simulink model "SWC_HALOUT_type"  (R2021b)
settings: Solver=FixedStepDiscrete  StartTime=0.0  StopTime=10.0  FixedStep=0.005  RelTol=1e-3
undefined symbols (not defined in the file): DIDLen_APPD, DIDLen_APPE, DIDLen_APPPedalZP, DIDLen_APSFunConfig, DIDLen_AutoLock, DIDLen_AutoWipHSpdEN, DIDLen_CALID, DIDLen_CDEODT, DIDLen_CLRDIST, DIDLen_DKCBLESta, DIDLen_DKCKey, DIDLen_DKCSta, DIDLen_DoorNFCAnchorSta, DIDLen_DRLDis, DIDLen_DynoMode, DIDLen_ECUNAME, DIDLen_FDDKCCoordXY, DIDLen_FMHTimer, DIDLen_LFLowPresThre, DIDLen_LFSensorID, DIDLen_LIDAAnchorSta, DIDLen_LRLowPresThre, DIDLen_LRSensorID, DIDLen_MILDIST, DIDLen_NUMPSATRIPSFLTMEMCLR, DIDLen_NVMPedalZP, DIDLen_OBDReq, DIDLen_ODOMETER, DIDLen_PKE, DIDLen_ProtocolId, DIDLen_PSA, DIDLen_QTYPSATRIPS, DIDLen_RFLowPresThre, DIDLen_RFSensorID, DIDLen_RRLowPresThre, DIDLen_RRSensorID, DIDLen_RUNTM, DIDLen_SensorMode, DIDLen_TestGroup, DIDLen_TireSize, DIDLen_TPMSLearnSta, DIDLen_TurnLampFLThreCurr, DIDLen_TurnLampFRThreCurr, DIDLen_TurnLampRLThreCurr, DIDLen_TurnLampRRThreCurr, DIDLen_UIDSta, DIDLen_USSConfig, DIDLen_UWBAnchorSta, DIDLen_VIN, DIDLen_VSS, DIDLen_WhlPres, DIDLen_WhlSensorBattSta, DIDLen_WhlTmp, DIDLen_WipRLSCmdCutFilter, DIDLen_WipRLSCmdHoldFilter, DIDLen_XWDMode, DIDNum_APPD, DIDNum_APPE, DIDNum_APPPedalZP, DIDNum_APSFunConfig ... (+504)
libraries: simulink x893, FVT_lib x320, hdlsllib x6, hcu_lib x5, halout x1
(part 5 of 11)

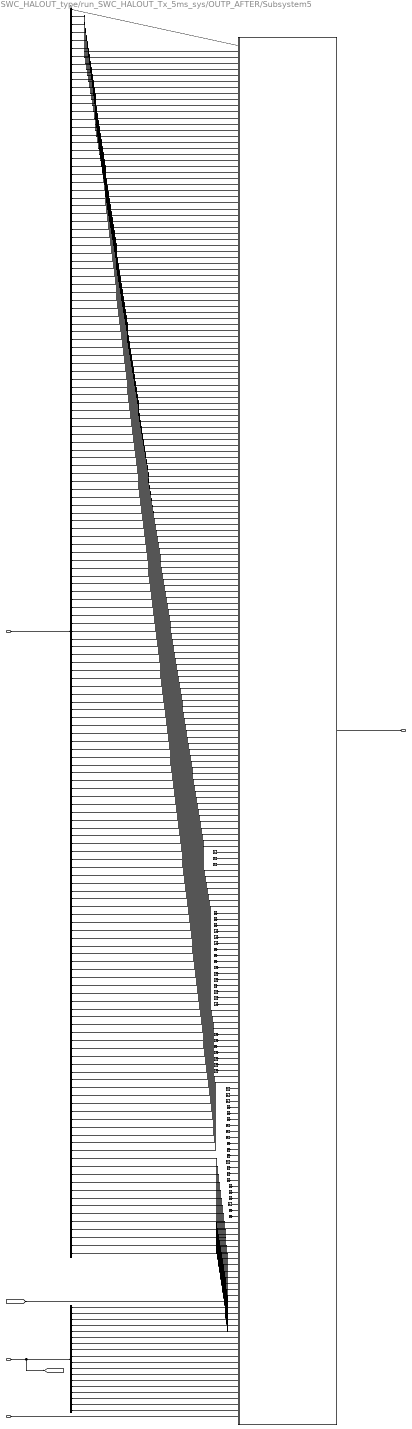
== system SWC_HALOUT_type/run_SWC_HALOUT_Tx_5ms_sys/OUTP_AFTER/Subsystem5 ==
  BOUTP_outputs : Inport
  BHAL_SYS_outputs : Inport  Port=2
  BHAL_DIDGetData_raw : Inport  Port=3
  Bus Selector : BusSelector  OutputSignals=VOUTP_AntitheftSta_enum,VOUTP_DrivetrainSelect_enum,VOUTP_WriteChkLFID_raw,VOUTP_WriteChkRFID_raw,VOUTP_WriteChkLRID_raw,VOUTP_WriteChkRRID_raw,VOUTP_WriteChkfinLFID_raw,VOUTP_WriteChkfinRFID_raw,VOUTP_WriteChkfinLRID_raw,VOUTP_WriteChkfinRRID_raw,VOUTP_LFSensorFail_flg,VOUTP_RFSensorFail_flg,VOUTP_LRSensorFail_flg,VOUTP_RRSensorFail_flg,VOUTP_LFWheelPSW_raw8,VOUTP_RFWheelPSW_raw8,VOUTP_LRWheelPSW_raw8,VOUTP_RRWheelPSW_raw8,VOUTP_LFPindi_enum,VOUTP_RFPind_enum,VOUTP_LRPindi_enum,VOUTP_RRPindi_enum,VOUTP_LFP20_raw8,VOUTP_RFP20_raw8,VOUTP_LRP20_raw8,VOUTP_RRP20_raw8,VOUTP_LFWheelPress_raw8,VOUTP_RFWheelPress_raw8,VOUTP_LRWheelPress_raw8,VOUTP_RRWheelPress_raw8,VOUTP_LFWheelTemp_C,VOUTP_RFWheelTemp_C,VOUTP_LRWheelTemp_C,VOUTP_RRWheelTemp_C,VOUTP_Flashchkdatavalid_enum,VOUTP_Flashdatavalid_enum,VOUTP_unlearnSfali_flg,VOUTP_unlearnSfailvalid_enum,VOUTP_Prepresstempvalid_enum,VOUTP_FlashS1ID_raw,VOUTP_FlashS2ID_raw,VOUTP_FlashS3ID_raw,VOUTP_FlashS4ID_raw,VOUTP_FlashIDvalid_enum,VOUTP_ACModeMem_enum,VOUTP_Face_flg,VOUTP_Foot_flg,VOUTP_Frost_flg,VOUTP_FaceM_flg,VOUTP_FootM_flg,VOUTP_CCUSyncSts_flg,VOUTP_ACForceOFF_flg,VOUTP_sigRecircSt_flg,VOUTP_RecAutoFlg_flg,VOUTP_AirIntenZone1M_enum,VOUTP_fdefog_flg,VOUTP_sigSetTempZon1St_C,VOUTP_sigSetTempZon2StM_C,VOUTP_CountAlarm_enum,VOUTP_MFSWTri_flg,VOUTP_MirrorFlodPos_flg,VOUTP_FuelDoorPos_flg,VOUTP_LockSettingStaMem_enum,VOUTP_MFRDNBrightReq_pct,VOUTP_RmLpModeENMem_enum,VOUTP_WiperFixMode_flg,VOUTP_SPTGENFunMem_enum,VOUTP_EAPS1MIN_pct,VOUTP_EAPS2MIN_pct,VOUTP_HoodSW_flg,VOUTP_TailgateSW_flg,VOUTP_CTDLockSW_flg,VOUTP_TailgateHDSW_flg,VOUTP_APMDoorControlSta_flg,VOUTP_fUnlockSingle_flg,VOUTP_SaveRegenMode_enum,VOUTP_AmbFunENFlash_enum,VOUTP_AmbWelENFlash_enum,VOUTP_AmbDimENFlash_enum,VOUTP_AmbLinkDriStaFlash_enum,VOUTP_AmbPwrWarnENFlash_enum,VOUTP_AmbODAENFlash_enum,VOUTP_AmbColorSta1_enum,VOUTP_AmbColorSta2_enum,VOUTP_AmbColorSta3_enum,VOUTP_AmbColorSta4_enum,VOUTP_AmbColorSta5_enum,VOUTP_AmbColorSta7_enum,VOUTP_AmbBrightnessSta1_enum,VOUTP_AmbBrightnessSta2_enum,VOUTP_AmbBrightnessSta3_enum,VOUTP_AmbBrightnessSta4_enum,VOUTP_AmbBrightnessSta5_enum,VOUTP_AmbBrightnessSta7_enum,VOUTP_TurnSwTimeSetSta123_enum,VOUTP_TurnSwTimeSetSta457_enum,VOUTP_FDCTHCAirIntZ3Sta_enum,VOUTP_FDCTHCREVentModeSta_enum,VOUTP_FDCTHCLEVentModeSta_enum,VOUTP_FDCTHCLEVentZSta_enum,VOUTP_FDCTHCCLEVentZSta_enum,VOUTP_FDCTHCREVentZSta_enum,VOUTP_FDCTHCCREVentZSta_enum,VOUTP_LVentEN_flg,VOUTP_FDCTHCLEVentYSta_enum,VOUTP_CLVentEN_flg,VOUTP_FDCTHCCLEVentYSta_enum,VOUTP_RVentEN_flg,VOUTP_FDCTHCREVentYSta_enum,VOUTP_CRVentEN_flg,VOUTP_FDCTHCCREVentYSta_enum,VOUTP_FDCFGSAirIntSta_enum,VOUTP_FDCFGSChSta_enum,VOUTP_FDCFGSIONSWSta_flg,VOUTP_WalkOutLkENMem_enum,VOUTP_WalkInUnLkENMem_enum,VOUTP_FollowMeENMem_enum,VOUTP_PTGUserHeight1_cnt,VOUTP_PTGUserHeight2_cnt,VOUTP_PTGUserHeight3_cnt,VOUTP_PTGUserHeight4_cnt,VOUTP_PTGUserHeight5_cnt,VOUTP_PTGUserHeight7_cnt,VOUTP_PTGOpenHeight12_enum,VOUTP_PTGOpenHeight34_enum,VOUTP_PTGOpenHeight57_enum,VOUTP_ACCLevelMem12_enum,VOUTP_ACCLevelMem34_enum,VOUTP_ACCLevelMem57_enum,VOUTP_AutoLockMem_enum,VOUTP_AutoUnlockMem_enum,VOUTP_MILDIST_km,VOUTP_CLRDIST_km,VOUTP_NUMPSATRIPSFLTMEMCLR_cnt,VOUTP_PSAR_sec,VOUTP_PSAL_sec,VOUTP_IPSAR_sec,VOUTP_IPSAL_sec,VOUTP_CPSAR_sec,VOUTP_CPSAL_sec,VOUTP_PKERNumerator_kphsqr,VOUTP_PKELNumerator_kphsqr,VOUTP_ODOMETER_km,VOUTP_ResetCDEODTR_km,VOUTP_QTYPSATRIPSR_cnt,VOUTP_QTYPSATRIPSL_cnt,VOUTP_HMIKey1FuncSta_enum,VOUTP_HMIKey2FuncSta_enum,VOUTP_HMIKey3FuncSta_enum,VOUTP_HMIKey4FuncSta_enum,VOUTP_HMIKey5FuncSta_enum,VOUTP_HMIKey6FuncSta_enum,VOUTP_HMIKey7FuncSta_enum,VOUTP_HMIKey8FuncSta_enum,VOUTP_AutoWipHSpdENSta_flg,VOUTP_ModelVersion_raw,VOUTP_ModelVersionChksum_raw,VOUTP_DIDModelVersion_raw,VOUTP_DIDModelVersionChksum_raw
  Bus Selector1 : BusSelector  OutputSignals=VHAL_RandomnumberY_raw1,VHAL_RandomnumberY_raw2,VHAL_RandomnumberY_raw3,VHAL_RandomnumberY_raw4,VHAL_RandomnumberY_raw5,VHAL_RandomnumberY_raw6,VHAL_RandomnumberY_raw7,VHAL_RandomnumberY_raw8,VHAL_funAuto_flg,VHAL_DiagDRLOFF_flg,VHAL_DiagFMHT_s,VHAL_DiagFLTC_mA,VHAL_DiagFRTC_mA,VHAL_DiagRLTC_mA,VHAL_DiagRRTC_mA,VHAL_USSConfig_raw8,VHAL_TireSize_raw8,VHAL_APSFunConfig_raw8
  Enabled Subsystem : Subsystem  TreatAsAtomicUnit=on
  Ground{,1..47} (48 alike) : Ground
  HAL_NvmWriteData_raw : Outport
  wires:
  BOUTP_outputs/1 -> Bus Selector/1
  Enabled Subsystem/1(HAL_NvmWriteData_raw) -> HAL_NvmWriteData_raw/1
  Bus Selector1/2 -> Enabled Subsystem/210(VHAL_RandomnumberY_raw2)  "<VHAL_RandomnumberY_raw2>"
  Bus Selector1/3 -> Enabled Subsystem/211(VHAL_RandomnumberY_raw3)  "<VHAL_RandomnumberY_raw3>"
  Bus Selector1/4 -> Enabled Subsystem/212(VHAL_RandomnumberY_raw4)  "<VHAL_RandomnumberY_raw4>"
  Bus Selector1/5 -> Enabled Subsystem/213(VHAL_RandomnumberY_raw5)  "<VHAL_RandomnumberY_raw5>"
  Bus Selector1/6 -> Enabled Subsystem/214(VHAL_RandomnumberY_raw6)  "<VHAL_RandomnumberY_raw6>"
  Bus Selector1/7 -> Enabled Subsystem/215(VHAL_RandomnumberY_raw7)  "<VHAL_RandomnumberY_raw7>"
  Bus Selector1/8 -> Enabled Subsystem/216(VHAL_RandomnumberY_raw8)  "<VHAL_RandomnumberY_raw8>"
  Bus Selector/24 -> Enabled Subsystem/24(VOUTP_RFP20_raw8)  "<VOUTP_RFP20_raw8>"
  Bus Selector/23 -> Enabled Subsystem/23(VOUTP_LFP20_raw8)  "<VOUTP_LFP20_raw8>"
  Bus Selector/25 -> Enabled Subsystem/25(VOUTP_LRP20_raw8)  "<VOUTP_LRP20_raw8>"
  Bus Selector/22 -> Enabled Subsystem/22(VOUTP_RRPindi_enum)  "<VOUTP_RRPindi_enum>"
  Bus Selector/26 -> Enabled Subsystem/26(VOUTP_RRP20_raw8)  "<VOUTP_RRP20_raw8>"
  Bus Selector/21 -> Enabled Subsystem/21(VOUTP_LRPindi_enum)  "<VOUTP_LRPindi_enum>"
  Bus Selector/27 -> Enabled Subsystem/27(VOUTP_LFWheelPress_raw8)  "<VOUTP_LFWheelPress_raw8>"
  Bus Selector/20 -> Enabled Subsystem/20(VOUTP_RFPindi_enum)  "<VOUTP_RFPind_enum>"
  Bus Selector/28 -> Enabled Subsystem/28(VOUTP_RFWheelPress_raw8)  "<VOUTP_RFWheelPress_raw8>"
  Bus Selector/19 -> Enabled Subsystem/19(VOUTP_LFPindi_enum)  "<VOUTP_LFPindi_enum>"
  Bus Selector/29 -> Enabled Subsystem/29(VOUTP_LRWheelPress_raw8)  "<VOUTP_LRWheelPress_raw8>"
  Bus Selector/56 -> Enabled Subsystem/56(VOUTP_fdefog_flg)  "<VOUTP_fdefog_flg>"
  Bus Selector/18 -> Enabled Subsystem/18(VOUTP_RRWheelPSW_raw8)  "<VOUTP_RRWheelPSW_raw8>"
  Bus Selector/30 -> Enabled Subsystem/30(VOUTP_RRWheelPress_raw8)  "<VOUTP_RRWheelPress_raw8>"
  Bus Selector/55 -> Enabled Subsystem/55(VOUTP_AirIntenZone1M_enum)  "<VOUTP_AirIntenZone1M_enum>"
  Bus Selector/17 -> Enabled Subsystem/17(VOUTP_LRWheelPSW_raw8)  "<VOUTP_LRWheelPSW_raw8>"
  Bus Selector/31 -> Enabled Subsystem/31(VOUTP_LFWheelTemp_C)  "<VOUTP_LFWheelTemp_C>"
  Bus Selector/54 -> Enabled Subsystem/54(VOUTP_RecAutoFlg_flg)  "<VOUTP_RecAutoFlg_flg>"
  Bus Selector/16 -> Enabled Subsystem/16(VOUTP_RFWheelPSW_raw8)  "<VOUTP_RFWheelPSW_raw8>"
  Bus Selector/32 -> Enabled Subsystem/32(VOUTP_RFWheelTemp_C)  "<VOUTP_RFWheelTemp_C>"
  Bus Selector/53 -> Enabled Subsystem/53(VOUTP_sigRecircSt_flg)  "<VOUTP_sigRecircSt_flg>"
  Bus Selector/15 -> Enabled Subsystem/15(VOUTP_LFWheelPSW_raw8)  "<VOUTP_LFWheelPSW_raw8>"
  Bus Selector/33 -> Enabled Subsystem/33(VOUTP_LRWheelTemp_C)  "<VOUTP_LRWheelTemp_C>"
  Bus Selector/52 -> Enabled Subsystem/52(VOUTP_ACForceOFF_flg)  "<VOUTP_ACForceOFF_flg>"
  Bus Selector/14 -> Enabled Subsystem/14(VOUTP_RRSensorFail_flg)  "<VOUTP_RRSensorFail_flg>"
  Bus Selector/34 -> Enabled Subsystem/34(VOUTP_RRWheelTemp_C)  "<VOUTP_RRWheelTemp_C>"
  Bus Selector/51 -> Enabled Subsystem/51(VOUTP_CCUSyncSts_flg)  "<VOUTP_CCUSyncSts_flg>"
  Bus Selector/13 -> Enabled Subsystem/13(VOUTP_LRSensorFail_flg)  "<VOUTP_LRSensorFail_flg>"
  Bus Selector/35 -> Enabled Subsystem/35(VOUTP_Flashchkdatavalid_enum)  "<VOUTP_Flashchkdatavalid_enum>"
  Bus Selector/50 -> Enabled Subsystem/50(VOUTP_FootM_flg)  "<VOUTP_FootM_flg>"
  Bus Selector/12 -> Enabled Subsystem/12(VOUTP_RFSensorFail_flg)  "<VOUTP_RFSensorFail_flg>"
  Bus Selector/36 -> Enabled Subsystem/36(VOUTP_Flashdatavalid_enum)  "<VOUTP_Flashdatavalid_enum>"
  Bus Selector/49 -> Enabled Subsystem/49(VOUTP_FaceM_flg)  "<VOUTP_FaceM_flg>"
  Bus Selector/11 -> Enabled Subsystem/11(VOUTP_LFSensorFail_flg)  "<VOUTP_LFSensorFail_flg>"
  Bus Selector/37 -> Enabled Subsystem/37(VOUTP_unlearnSfali_flg)  "<VOUTP_unlearnSfali_flg>"
  Bus Selector/48 -> Enabled Subsystem/48(VOUTP_Frost_flg)  "<VOUTP_Frost_flg>"
  Bus Selector/38 -> Enabled Subsystem/38(VOUTP_unlearnSfailvalid_enum)  "<VOUTP_unlearnSfailvalid_enum>"
  Bus Selector/47 -> Enabled Subsystem/47(VOUTP_Foot_flg)  "<VOUTP_Foot_flg>"
  Bus Selector/39 -> Enabled Subsystem/39(VOUTP_Prepresstempvalid_enum)  "<VOUTP_Prepresstempvalid_enum>"
  Bus Selector/46 -> Enabled Subsystem/46(VOUTP_Face_flg)  "<VOUTP_Face_flg>"
  Bus Selector/2 -> Enabled Subsystem/2(VOUTP_DrivetrainSelect_enum)  "<VOUTP_DrivetrainSelect_enum>"
  Bus Selector/1 -> Enabled Subsystem/1(VOUTP_AntitheftSta_enum)  "<VOUTP_AntitheftSta_enum>"
  Bus Selector/10 -> Enabled Subsystem/10(VOUTP_WriteChkfinRRID_raw)  "<VOUTP_WriteChkfinRRID_raw>"
  Bus Selector/9 -> Enabled Subsystem/9(VOUTP_WriteChkfinLRID_raw)  "<VOUTP_WriteChkfinLRID_raw>"
  Bus Selector/8 -> Enabled Subsystem/8(VOUTP_WriteChkfinRFID_raw)  "<VOUTP_WriteChkfinRFID_raw>"
  Bus Selector/7 -> Enabled Subsystem/7(VOUTP_WriteChkfinLFID_raw)  "<VOUTP_WriteChkfinLFID_raw>"
  Bus Selector/6 -> Enabled Subsystem/6(VOUTP_WriteChkRRID_raw)  "<VOUTP_WriteChkRRID_raw>"
  Bus Selector/5 -> Enabled Subsystem/5(VOUTP_WriteChkLRID_raw)  "<VOUTP_WriteChkLRID_raw>"
  Bus Selector/4 -> Enabled Subsystem/4(VOUTP_WriteChkRFID_raw)  "<VOUTP_WriteChkRFID_raw>"
  Bus Selector/3 -> Enabled Subsystem/3(VOUTP_WriteChkLFID_raw)  "<VOUTP_WriteChkLFID_raw>"
  Bus Selector/58 -> Enabled Subsystem/58(VOUTP_sigSetTempZon2StM_C)  "<VOUTP_sigSetTempZon2StM_C>"
  Bus Selector/59 -> Enabled Subsystem/59(VOUT_CountAlarm_enum)  "<VOUTP_CountAlarm_enum>"
  Bus Selector/57 -> Enabled Subsystem/57(VOUTP_sigSetTempZon1St_C)  "<VOUTP_sigSetTempZon1St_C>"
  Bus Selector/60 -> Enabled Subsystem/60(VOUTP_MFSWTri_flg)  "<VOUTP_MFSWTri_flg>"
  Bus Selector/61 -> Enabled Subsystem/61(VOUTP_MirrorFlodPos_flg)  "<VOUTP_MirrorFlodPos_flg>"
  Bus Selector/62 -> Enabled Subsystem/62(VOUTP_FuelDoorPos_flg)  "<VOUTP_FuelDoorPos_flg>"
  Bus Selector/63 -> Enabled Subsystem/63(VOUTP_LockSetting_flg)  "<VOUTP_LockSettingStaMem_enum>"
  Bus Selector/64 -> Enabled Subsystem/64(VOUTP_MFRDNBrightReq_pct)  "<VOUTP_MFRDNBrightReq_pct>"
  Bus Selector/65 -> Enabled Subsystem/65(VOUTP_RoomLampMode_flg)  "<VOUTP_RmLpModeENMem_enum>"
  Bus Selector/66 -> Enabled Subsystem/66(VOUTP_WiperFixMode_flg)  "<VOUTP_WiperFixMode_flg>"
  Bus Selector/67 -> Enabled Subsystem/67(VOUTP_IVIPTGUSStaSW_flg)  "<VOUTP_SPTGENFunMem_enum>"
  Bus Selector1/1 -> Enabled Subsystem/209(VHAL_RandomnumberY_raw1)  "<VHAL_RandomnumberY_raw1>"
  Bus Selector/45 -> Enabled Subsystem/45(VOUTP_ACModeMem_enum)  "<VOUTP_ACModeMem_enum>"
  Bus Selector/40 -> Enabled Subsystem/40(VOUTP_FlashS1ID_raw)  "<VOUTP_FlashS1ID_raw>"
  Bus Selector/41 -> Enabled Subsystem/41(VOUTP_FlashS2ID_raw)  "<VOUTP_FlashS2ID_raw>"
  Bus Selector/42 -> Enabled Subsystem/42(VOUTP_FlashS3ID_raw)  "<VOUTP_FlashS3ID_raw>"
  Bus Selector/43 -> Enabled Subsystem/43(VOUTP_FlashS41ID_raw)  "<VOUTP_FlashS4ID_raw>"
  Bus Selector/44 -> Enabled Subsystem/44(VOUTP_FlashIDvalid_enum)  "<VOUTP_FlashIDvalid_enum>"
  BHAL_SYS_outputs/1 -> [BHAL_SYS_outputs], Bus Selector1/1
  Bus Selector/68 -> Enabled Subsystem/68(VOUTP_EAPS1MIN_pct)  "<VOUTP_EAPS1MIN_pct>"
  Bus Selector/69 -> Enabled Subsystem/69(VOUTP_EAPS2MIN_pct)  "<VOUTP_EAPS2MIN_pct>"
  Bus Selector/70 -> Enabled Subsystem/70(VOUTP_HoodSW_flg)  "<VOUTP_HoodSW_flg>"
  Bus Selector/71 -> Enabled Subsystem/71(VOUTP_TailgateSW_flg)  "<VOUTP_TailgateSW_flg>"
  Bus Selector/72 -> Enabled Subsystem/72(VOUTP_CTDLockSW_flg)  "<VOUTP_CTDLockSW_flg>"
  Bus Selector/73 -> Enabled Subsystem/73(VOUTP_TailgateHDSW_flg)  "<VOUTP_TailgateHDSW_flg>"
  Bus Selector/74 -> Enabled Subsystem/74(VOUTP_APMDoorControlSta_flg)  "<VOUTP_APMDoorControlSta_flg>"
  Bus Selector1/9 -> Enabled Subsystem/217(VHAL_funAuto_flg)  "<VHAL_funAuto_flg>"
  Bus Selector1/10 -> Enabled Subsystem/218(VHAL_DiagDRLOFF_flg)  "<VHAL_DiagDRLOFF_flg>"
  Bus Selector1/11 -> Enabled Subsystem/219(VHAL_DiagFMHT_s)  "<VHAL_DiagFMHT_s>"
  Bus Selector1/12 -> Enabled Subsystem/220(VHAL_DiagFLTC_mA)  "<VHAL_DiagFLTC_mA>"
  Bus Selector1/13 -> Enabled Subsystem/221(VHAL_DiagFRTC_mA)  "<VHAL_DiagFRTC_mA>"
  Bus Selector1/14 -> Enabled Subsystem/222(VHAL_DiagRLTC_mA)  "<VHAL_DiagRLTC_mA>"
  Bus Selector1/15 -> Enabled Subsystem/223(VHAL_DiagRRTC_mA)  "<VHAL_DiagRRTC_mA>"
  Bus Selector1/16 -> Enabled Subsystem/224(VHAL_USSConfig_raw8)  "<VHAL_USSConfig_raw8>"
  Bus Selector1/17 -> Enabled Subsystem/225(VHAL_TireSize_raw8)  "<VHAL_TireSize_raw8>"
  Bus Selector1/18 -> Enabled Subsystem/226(VHAL_APSFunConfig_raw8)  "<VHAL_APSFunConfig_raw8>"
  Bus Selector/75 -> Enabled Subsystem/75(VOUTP_fUnlockSingle_flg)  "<VOUTP_fUnlockSingle_flg>"
  Bus Selector/76 -> Enabled Subsystem/76(VOUTP_SaveRegenMode_enum)  "<VOUTP_SaveRegenMode_enum>"
  Bus Selector/77 -> Enabled Subsystem/77(VOUTP_AmbFunENFlash_enum)  "<VOUTP_AmbFunENFlash_enum>"
  Bus Selector/78 -> Enabled Subsystem/78(VOUTP_AmbWelENFlash_enum)  "<VOUTP_AmbWelENFlash_enum>"
  Bus Selector/79 -> Enabled Subsystem/79(VOUTP_AmbDimENFlash_enum)  "<VOUTP_AmbDimENFlash_enum>"
  Bus Selector/80 -> Enabled Subsystem/80(VOUTP_AmbLinkDriStaFlash_enum)  "<VOUTP_AmbLinkDriStaFlash_enum>"
  Bus Selector/81 -> Enabled Subsystem/81(VOUTP_AmbPwrWarnENFlash_enum)  "<VOUTP_AmbPwrWarnENFlash_enum>"
  Bus Selector/82 -> Enabled Subsystem/82(VOUTP_AmbODAENFlash_enum)  "<VOUTP_AmbODAENFlash_enum>"
  Bus Selector/83 -> Enabled Subsystem/83(VOUTP_AmbColorSta1_enum)  "<VOUTP_AmbColorSta1_enum>"
  Bus Selector/84 -> Enabled Subsystem/84(VOUTP_AmbColorSta2_enum)  "<VOUTP_AmbColorSta2_enum>"
  Bus Selector/85 -> Enabled Subsystem/85(VOUTP_AmbColorSta3_enum)  "<VOUTP_AmbColorSta3_enum>"
  Bus Selector/86 -> Enabled Subsystem/86(VOUTP_AmbColorSta4_enum)  "<VOUTP_AmbColorSta4_enum>"
  Bus Selector/87 -> Enabled Subsystem/87(VOUTP_AmbColorSta5_enum)  "<VOUTP_AmbColorSta5_enum>"
  Bus Selector/88 -> Enabled Subsystem/88(VOUTP_AmbColorSta7_enum)  "<VOUTP_AmbColorSta7_enum>"
  Bus Selector/89 -> Enabled Subsystem/89(VOUTP_AmbBrightnessSta1_enum)  "<VOUTP_AmbBrightnessSta1_enum>"
  Bus Selector/90 -> Enabled Subsystem/90(VOUTP_AmbBrightnessSta2_enum)  "<VOUTP_AmbBrightnessSta2_enum>"
  Bus Selector/91 -> Enabled Subsystem/91(VOUTP_AmbBrightnessSta3_enum)  "<VOUTP_AmbBrightnessSta3_enum>"
  Bus Selector/92 -> Enabled Subsystem/92(VOUTP_AmbBrightnessSta4_enum)  "<VOUTP_AmbBrightnessSta4_enum>"
  Bus Selector/93 -> Enabled Subsystem/93(VOUTP_AmbBrightnessSta5_enum)  "<VOUTP_AmbBrightnessSta5_enum>"
  Bus Selector/94 -> Enabled Subsystem/94(VOUTP_AmbBrightnessSta7_enum)  "<VOUTP_AmbBrightnessSta7_enum>"
  Bus Selector/95 -> Enabled Subsystem/95(VOUTP_TurnSwTimeSetSta123_enum)  "<VOUTP_TurnSwTimeSetSta123_enum>"
  Bus Selector/96 -> Enabled Subsystem/96(VOUTP_TurnSwTimeSetSta457_enum)  "<VOUTP_TurnSwTimeSetSta457_enum>"
  Bus Selector/97 -> Enabled Subsystem/97(VOUTP_FDCTHCAirIntZ3Sta_enum)  "<VOUTP_FDCTHCAirIntZ3Sta_enum>"
  Bus Selector/98 -> Enabled Subsystem/98(VOUTP_FDCTHCREVentModeSta_enum)  "<VOUTP_FDCTHCREVentModeSta_enum>"
  Bus Selector/99 -> Enabled Subsystem/99(VOUTP_FDCTHCLEVentModeSta_enum)  "<VOUTP_FDCTHCLEVentModeSta_enum>"
  Bus Selector/100 -> Enabled Subsystem/100(VOUTP_FDCTHCLEVentZSta_enum)  "<VOUTP_FDCTHCLEVentZSta_enum>"
  Bus Selector/101 -> Enabled Subsystem/101(VOUTP_FDCTHCCLEVentZSta_enum)  "<VOUTP_FDCTHCCLEVentZSta_enum>"
  Bus Selector/102 -> Enabled Subsystem/102(VOUTP_FDCTHCREVentZSta_enum)  "<VOUTP_FDCTHCREVentZSta_enum>"
  Bus Selector/103 -> Enabled Subsystem/103(VOUTP_FDCTHCCREVentZSta_enum)  "<VOUTP_FDCTHCCREVentZSta_enum>"
  Bus Selector/104 -> Enabled Subsystem/104(VOUTP_LVentEN_flg)  "<VOUTP_LVentEN_flg>"
  Bus Selector/105 -> Enabled Subsystem/105(VOUTP_FDCTHCLEVentYSta_enum)  "<VOUTP_FDCTHCLEVentYSta_enum>"
  Bus Selector/106 -> Enabled Subsystem/106(VOUTP_CLVentEN_flg)  "<VOUTP_CLVentEN_flg>"
  Bus Selector/107 -> Enabled Subsystem/107(VOUTP_FDCTHCCLEVentYSta_enum)  "<VOUTP_FDCTHCCLEVentYSta_enum>"
  Bus Selector/108 -> Enabled Subsystem/108(VOUTP_RVentEN_flg)  "<VOUTP_RVentEN_flg>"
  Bus Selector/109 -> Enabled Subsystem/109(VOUTP_FDCTHCREVentYSta_enum)  "<VOUTP_FDCTHCREVentYSta_enum>"
  Bus Selector/110 -> Enabled Subsystem/110(VOUTP_CRVentEN_flg)  "<VOUTP_CRVentEN_flg>"
  Bus Selector/111 -> Enabled Subsystem/111(VOUTP_FDCTHCCREVentYSta_enum)  "<VOUTP_FDCTHCCREVentYSta_enum>"
  Bus Selector/112 -> Enabled Subsystem/112(VOUTP_FDCFGSAirIntSta_enum)  "<VOUTP_FDCFGSAirIntSta_enum>"
  Bus Selector/113 -> Enabled Subsystem/113(VOUTP_FDCFGSChSta_enum)  "<VOUTP_FDCFGSChSta_enum>"
  Bus Selector/114 -> Enabled Subsystem/114(VOUTP_FDCFGSIONSWSta_flg)  "<VOUTP_FDCFGSIONSWSta_flg>"
  Bus Selector/115 -> Enabled Subsystem/115(VOUTP_WalkOutLkENFunSta_flg)  "<VOUTP_WalkOutLkENMem_enum>"
  Bus Selector/116 -> Enabled Subsystem/116(VOUTP_WalkInUnLkENFunSta_flg)  "<VOUTP_WalkInUnLkENMem_enum>"
  Bus Selector/117 -> Enabled Subsystem/117(VOUTP_FollowMeENFunSta_flg)  "<VOUTP_FollowMeENMem_enum>"
  Bus Selector/118 -> Enabled Subsystem/118(VOUTP_PTGUserHeight1_cnt)  "<VOUTP_PTGUserHeight1_cnt>"
  Bus Selector/119 -> Enabled Subsystem/119(VOUTP_PTGUserHeight2_cnt)  "<VOUTP_PTGUserHeight2_cnt>"
  Bus Selector/120 -> Enabled Subsystem/120(VOUTP_PTGUserHeight3_cnt)  "<VOUTP_PTGUserHeight3_cnt>"
  Bus Selector/121 -> Enabled Subsystem/121(VOUTP_PTGUserHeight4_cnt)  "<VOUTP_PTGUserHeight4_cnt>"
  Bus Selector/122 -> Enabled Subsystem/122(VOUTP_PTGUserHeight5_cnt)  "<VOUTP_PTGUserHeight5_cnt>"
  Bus Selector/123 -> Enabled Subsystem/123(VOUTP_PTGUserHeight7_cnt)  "<VOUTP_PTGUserHeight7_cnt>"
  Bus Selector/124 -> Enabled Subsystem/124(VOUTP_PTGOpenHeight12_enum)  "<VOUTP_PTGOpenHeight12_enum>"
  Bus Selector/125 -> Enabled Subsystem/125(VOUTP_PTGOpenHeight34_enum)  "<VOUTP_PTGOpenHeight34_enum>"
  Bus Selector/126 -> Enabled Subsystem/126(VOUTP_PTGOpenHeight57_enum)  "<VOUTP_PTGOpenHeight57_enum>"
  BHAL_DIDGetData_raw/1 -> Enabled Subsystem/227(BHAL_DIDGetData_raw)
  Bus Selector/127 -> Enabled Subsystem/127(VOUTP_ACCLevelMem12_enum)  "<VOUTP_ACCLevelMem12_enum>"
  Bus Selector/128 -> Enabled Subsystem/128(VOUTP_ACCLevelMem34_enum)  "<VOUTP_ACCLevelMem34_enum>"
  Bus Selector/129 -> Enabled Subsystem/129(VOUTP_ACCLevelMem57_enum)  "<VOUTP_ACCLevelMem57_enum>"
  Bus Selector/130 -> Enabled Subsystem/130(VOUTP_AutoLockMem_enum)  "<VOUTP_AutoLockMem_enum>"
  Bus Selector/131 -> Enabled Subsystem/131(VOUTP_AutoUnlockMem_enum)  "<VOUTP_AutoUnlockMem_enum>"
  Bus Selector/132 -> Enabled Subsystem/132(VOUTP_MILDIST_km)  "<VOUTP_MILDIST_km>"
  Bus Selector/133 -> Enabled Subsystem/133(VOUTP_CLRDIST_km)  "<VOUTP_CLRDIST_km>"
  Bus Selector/134 -> Enabled Subsystem/137(VOUTP_NUMPSATRIPSFLTMEMCLR_cnt)  "<VOUTP_NUMPSATRIPSFLTMEMCLR_cnt>"
  Bus Selector/135 -> Enabled Subsystem/138(VOUTP_PSAR_sec)  "<VOUTP_PSAR_sec>"
  Bus Selector/136 -> Enabled Subsystem/139(VOUTP_PSAL_sec)  "<VOUTP_PSAL_sec>"
  Bus Selector/137 -> Enabled Subsystem/140(VOUTP_IPSAR_sec)  "<VOUTP_IPSAR_sec>"
  Bus Selector/138 -> Enabled Subsystem/141(VOUTP_IPSAL_sec)  "<VOUTP_IPSAL_sec>"
  Bus Selector/139 -> Enabled Subsystem/142(VOUTP_CPSAR_sec)  "<VOUTP_CPSAR_sec>"
  Bus Selector/140 -> Enabled Subsystem/143(VOUTP_CPSAL_sec)  "<VOUTP_CPSAL_sec>"
  Bus Selector/143 -> Enabled Subsystem/162(VOUTP_ODOMETER_km)  "<VOUTP_ODOMETER_km>"
  Bus Selector/145 -> Enabled Subsystem/171(VOUTP_QTYPSATRIPSR_cnt)  "<VOUTP_QTYPSATRIPSR_cnt>"
  Bus Selector/146 -> Enabled Subsystem/172(VOUTP_QTYPSATRIPSL_cnt)  "<VOUTP_QTYPSATRIPSL_cnt>"
  Bus Selector/144 -> Enabled Subsystem/163(VOUTP_ResetCDEODTR_km)  "<VOUTP_ResetCDEODTR_km>"
  Bus Selector/141 -> Enabled Subsystem/160(VOUTP_PKERNumerator_kphsqr)  "<VOUTP_PKERNumerator_kphsqr>"
  Bus Selector/142 -> Enabled Subsystem/161(VOUTP_PKELNumerator_kphsqr)  "<VOUTP_PKELNumerator_kphsqr>"
  [BHAL_SYS_outputs] -> Enabled Subsystem/208(BHAL_SYS_outputs)
  Bus Selector/147 -> Enabled Subsystem/195(VOUTP_HMIKey1FuncSta_enum)  "<VOUTP_HMIKey1FuncSta_enum>"
  Bus Selector/148 -> Enabled Subsystem/196(VOUTP_HMIKey2FuncSta_enum)  "<VOUTP_HMIKey2FuncSta_enum>"
  Bus Selector/149 -> Enabled Subsystem/197(VOUTP_HMIKey3FuncSta_enum)  "<VOUTP_HMIKey3FuncSta_enum>"
  Bus Selector/150 -> Enabled Subsystem/198(VOUTP_HMIKey4FuncSta_enum)  "<VOUTP_HMIKey4FuncSta_enum>"
  Bus Selector/151 -> Enabled Subsystem/199(VOUTP_HMIKey5FuncSta_enum)  "<VOUTP_HMIKey5FuncSta_enum>"
  Bus Selector/152 -> Enabled Subsystem/200(VOUTP_HMIKey6FuncSta_enum)  "<VOUTP_HMIKey6FuncSta_enum>"
  Bus Selector/153 -> Enabled Subsystem/201(VOUTP_HMIKey7FuncSta_enum)  "<VOUTP_HMIKey7FuncSta_enum>"
  Bus Selector/154 -> Enabled Subsystem/202(VOUTP_HMIKey8FuncSta_enum)  "<VOUTP_HMIKey8FuncSta_enum>"
  Bus Selector/155 -> Enabled Subsystem/203(VOUTP_AutoWipHSpdENSta_flg)  "<VOUTP_AutoWipHSpdENSta_flg>"
  Bus Selector/156 -> Enabled Subsystem/204(VOUTP_ModelVersion_raw)  "<VOUTP_ModelVersion_raw>"
  Bus Selector/157 -> Enabled Subsystem/205(VOUTP_ModelVersionChksum_raw)  "<VOUTP_ModelVersionChksum_raw>"
  Bus Selector/158 -> Enabled Subsystem/206(VOUTP_DIDModelVersion_raw)  "<VOUTP_DIDModelVersion_raw>"
  Bus Selector/159 -> Enabled Subsystem/207(VOUTP_DIDModelVersionChksum_raw)  "<VOUTP_DIDModelVersionChksum_raw>"
  Ground/1 -> Enabled Subsystem/134(VOUTP_WARMUPS_cnt)
  Ground1/1 -> Enabled Subsystem/135(VOUTP_MILTIME_min)
  Ground2/1 -> Enabled Subsystem/136(VOUTP_CLRTIME_min)
  Ground4/1 -> Enabled Subsystem/145(VOUTP_IGNCNTR_cnt)
  Ground5/1 -> Enabled Subsystem/146(VOUTP_TNBCPSAR_Ahr)
  Ground3/1 -> Enabled Subsystem/144(VOUTP_HVBNAH_Ahr)
  Ground6/1 -> Enabled Subsystem/147(VOUTP_TNBCPSAL_Ahr)
  Ground8/1 -> Enabled Subsystem/149(VOUTP_TNECPSAL_kWh)
  Ground7/1 -> Enabled Subsystem/148(VOUTP_TNECPSAR_kWh)
  Ground13/1 -> Enabled Subsystem/154(VOUTP_GECHGOVCDCR_kWh)
  Ground14/1 -> Enabled Subsystem/155(VOUTP_GECHGOVCDCL_kWh)
  Ground12/1 -> Enabled Subsystem/153(VOUTP_TGEOVCL_kWh)
  Ground9/1 -> Enabled Subsystem/150(VOUTP_TEBPSAR_kWh)
  Ground11/1 -> Enabled Subsystem/152(VOUTP_TGEOVCR_kWh)
  Ground10/1 -> Enabled Subsystem/151(VOUTP_TEBPSAL_kWh)
  Ground15/1 -> Enabled Subsystem/156(VOUTP_GECHGOVCACR_kWh)
  Ground16/1 -> Enabled Subsystem/157(VOUTP_GECHGOVCACL_kWh)
  Ground18/1 -> Enabled Subsystem/159(VOUTP_RESSV2XENNONPSAL_kWh)
  Ground17/1 -> Enabled Subsystem/158(VOUTP_RESSV2XENNONPSAR_kWh)
  Ground19/1 -> Enabled Subsystem/164(VOUTP_AvgBattTempPSAR_C)
  Ground23/1 -> Enabled Subsystem/168(VOUTP_AvgBattTempOFFR_C)
  Ground24/1 -> Enabled Subsystem/169(VOUTP_AvgBattTempOFFL_C)
  Ground20/1 -> Enabled Subsystem/165(VOUTP_AvgBattTempPSAL_C)
  Ground22/1 -> Enabled Subsystem/167(VOUTP_AvgBattTempOVCL_C)
  Ground21/1 -> Enabled Subsystem/166(VOUTP_AvgBattTempOVCR_C)
  Ground25/1 -> Enabled Subsystem/170(VOUTP_HVBNE_kWh)
  Ground27/1 -> Enabled Subsystem/181(VOUTP_RESSTIMESOCCHGRNGR_s)
  Ground41/1 -> Enabled Subsystem/179(VOUTP_RESSTIMESOCPSARNGR_s)
  Ground26/1 -> Enabled Subsystem/180(VOUTP_RESSTIMESOCPSARNGL_s)
  Ground28/1 -> Enabled Subsystem/182(VOUTP_RESSTIMESOCOFFRNGL_s)
  Ground29/1 -> Enabled Subsystem/183(VOUTP_MAXBATTEMPL_C)
  Ground36/1 -> Enabled Subsystem/174(VOUTP_ETMBTOER_kWh)
  Ground37/1 -> Enabled Subsystem/175(VOUTP_ETMBTOEL_kWh)
  Ground34/1 -> Enabled Subsystem/188(VOUTP_AVGBATTEMPL_C)
  Ground30/1 -> Enabled Subsystem/184(VOUTP_MINBATTEMPL_C)
  Ground35/1 -> Enabled Subsystem/173(VOUTP_RESSCNTDODRNGR_cnt)
  Ground31/1 -> Enabled Subsystem/185(VOUTP_RESSTIMESOCCHGRNGL_s)
  Ground38/1 -> Enabled Subsystem/176(VOUTP_RESSCNTDODRNGL_cnt)
  Ground33/1 -> Enabled Subsystem/187(VOUTP_AVGBATTEMPL_sec)
  Ground40/1 -> Enabled Subsystem/178(VOUTP_ETMATOEL_kWh)
  Ground32/1 -> Enabled Subsystem/186(VOUTP_RESSTIMESOCOFFRNGR_s)
  Ground39/1 -> Enabled Subsystem/177(VOUTP_ETMATOER_kWh)
  Ground46/1 -> Enabled Subsystem/193(VOUTP_OFFR_sec)
  Ground47/1 -> Enabled Subsystem/194(VOUTP_OFFL_sec)
  Ground45/1 -> Enabled Subsystem/192(VOUTP_OVCL_sec)
  Ground44/1 -> Enabled Subsystem/191(VOUTP_OVCR_sec)
  Ground43/1 -> Enabled Subsystem/190(VOUTP_BattTempPSAL_sec)
  Ground42/1 -> Enabled Subsystem/189(VOUTP_BattTempPSAR_sec)

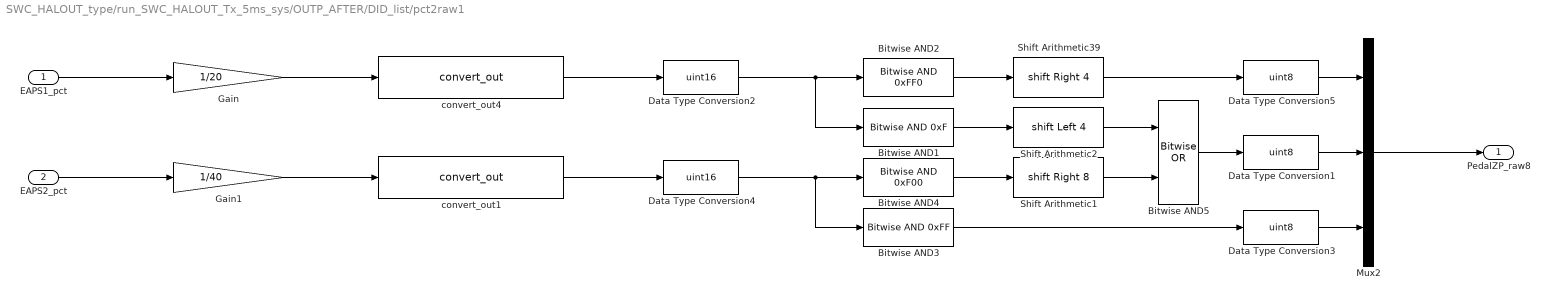
== system SWC_HALOUT_type/run_SWC_HALOUT_Tx_5ms_sys/OUTP_AFTER/DID_list/pct2raw1 ==
  EAPS1_pct : Inport
  EAPS2_pct : Inport  Port=2
  Bitwise AND1 : simulink/Logic and Bit Operations/Bitwise Operator  logicop=AND  UseBitMask=on  BitMask=0xF  BitMaskRealWorld=Stored Integer
  Bitwise AND2 : simulink/Logic and Bit Operations/Bitwise Operator  logicop=AND  UseBitMask=on  BitMask=0xFF0  BitMaskRealWorld=Stored Integer
  Bitwise AND3 : simulink/Logic and Bit Operations/Bitwise Operator  logicop=AND  UseBitMask=on  BitMask=0xFF  BitMaskRealWorld=Stored Integer
  Bitwise AND4 : simulink/Logic and Bit Operations/Bitwise Operator  logicop=AND  UseBitMask=on  BitMask=0xF00  BitMaskRealWorld=Stored Integer
  Bitwise AND5 : simulink/Logic and Bit Operations/Bitwise Operator  logicop=OR  UseBitMask=off  NumInputPorts=2  BitMask=0xFF  BitMaskRealWorld=Stored Integer
  Data Type Conversion1 : DataTypeConversion  OutDataTypeStr=uint8
  Data Type Conversion2 : DataTypeConversion  OutDataTypeStr=uint16
  Data Type Conversion3 : DataTypeConversion  OutDataTypeStr=uint8
  Data Type Conversion4 : DataTypeConversion  OutDataTypeStr=uint16
  Data Type Conversion5 : DataTypeConversion  OutDataTypeStr=uint8
  Gain : Gain  Gain=1/20
  Gain1 : Gain  Gain=1/40
  Mux2 : Mux  Inputs=3
  Shift Arithmetic1 : ArithShift  BitShiftNumber=8  BitShiftDirection=Right
  Shift Arithmetic2 : ArithShift  BitShiftNumber=4  BitShiftDirection=Left
  Shift Arithmetic39 : ArithShift  BitShiftNumber=4  BitShiftDirection=Right
  convert_out1 : FVT_lib/hal/convert_out  gain=0.001  offset=0
  convert_out4 : FVT_lib/hal/convert_out  gain=0.001  offset=0
  PedalZP_raw8 : Outport
  wires:
  Data Type Conversion1/1 -> Mux2/2
  Bitwise AND5/1 -> Data Type Conversion1/1
  Shift Arithmetic1/1 -> Bitwise AND5/2
  Shift Arithmetic2/1 -> Bitwise AND5/1
  Gain1/1 -> convert_out1/1
  Gain/1 -> convert_out4/1
  EAPS1_pct/1 -> Gain/1
  convert_out4/1 -> Data Type Conversion2/1
  convert_out1/1 -> Data Type Conversion4/1
  EAPS2_pct/1 -> Gain1/1
  Bitwise AND3/1 -> Data Type Conversion3/1
  Bitwise AND4/1 -> Shift Arithmetic1/1
  Data Type Conversion4/1 -> Bitwise AND3/1, Bitwise AND4/1
  Data Type Conversion3/1 -> Mux2/3
  Data Type Conversion5/1 -> Mux2/1
  Data Type Conversion2/1 -> Bitwise AND2/1, Bitwise AND1/1
  Bitwise AND2/1 -> Shift Arithmetic39/1
  Shift Arithmetic39/1 -> Data Type Conversion5/1
  Mux2/1 -> PedalZP_raw8/1
  Bitwise AND1/1 -> Shift Arithmetic2/1

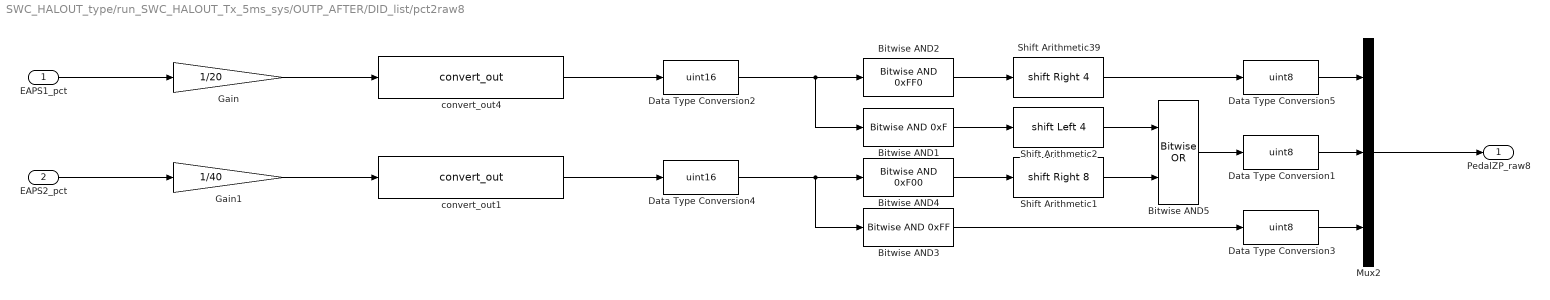
== system SWC_HALOUT_type/run_SWC_HALOUT_Tx_5ms_sys/OUTP_AFTER/DID_list/pct2raw8 ==
  EAPS1_pct : Inport
  EAPS2_pct : Inport  Port=2
  Bitwise AND1 : simulink/Logic and Bit Operations/Bitwise Operator  logicop=AND  UseBitMask=on  BitMask=0xF  BitMaskRealWorld=Stored Integer
  Bitwise AND2 : simulink/Logic and Bit Operations/Bitwise Operator  logicop=AND  UseBitMask=on  BitMask=0xFF0  BitMaskRealWorld=Stored Integer
  Bitwise AND3 : simulink/Logic and Bit Operations/Bitwise Operator  logicop=AND  UseBitMask=on  BitMask=0xFF  BitMaskRealWorld=Stored Integer
  Bitwise AND4 : simulink/Logic and Bit Operations/Bitwise Operator  logicop=AND  UseBitMask=on  BitMask=0xF00  BitMaskRealWorld=Stored Integer
  Bitwise AND5 : simulink/Logic and Bit Operations/Bitwise Operator  logicop=OR  UseBitMask=off  NumInputPorts=2  BitMask=0xFF  BitMaskRealWorld=Stored Integer
  Data Type Conversion1 : DataTypeConversion  OutDataTypeStr=uint8
  Data Type Conversion2 : DataTypeConversion  OutDataTypeStr=uint16
  Data Type Conversion3 : DataTypeConversion  OutDataTypeStr=uint8
  Data Type Conversion4 : DataTypeConversion  OutDataTypeStr=uint16
  Data Type Conversion5 : DataTypeConversion  OutDataTypeStr=uint8
  Gain : Gain  Gain=1/20
  Gain1 : Gain  Gain=1/40
  Mux2 : Mux  Inputs=3
  Shift Arithmetic1 : ArithShift  BitShiftNumber=8  BitShiftDirection=Right
  Shift Arithmetic2 : ArithShift  BitShiftNumber=4  BitShiftDirection=Left
  Shift Arithmetic39 : ArithShift  BitShiftNumber=4  BitShiftDirection=Right
  convert_out1 : FVT_lib/hal/convert_out  gain=0.001  offset=0
  convert_out4 : FVT_lib/hal/convert_out  gain=0.001  offset=0
  PedalZP_raw8 : Outport
  wires:
  Bitwise AND1/1 -> Shift Arithmetic2/1
  Mux2/1 -> PedalZP_raw8/1
  Shift Arithmetic39/1 -> Data Type Conversion5/1
  Bitwise AND2/1 -> Shift Arithmetic39/1
  Data Type Conversion2/1 -> Bitwise AND1/1, Bitwise AND2/1
  Data Type Conversion5/1 -> Mux2/1
  Data Type Conversion3/1 -> Mux2/3
  Data Type Conversion4/1 -> Bitwise AND4/1, Bitwise AND3/1
  Bitwise AND4/1 -> Shift Arithmetic1/1
  Bitwise AND3/1 -> Data Type Conversion3/1
  EAPS2_pct/1 -> Gain1/1
  convert_out1/1 -> Data Type Conversion4/1
  convert_out4/1 -> Data Type Conversion2/1
  EAPS1_pct/1 -> Gain/1
  Gain/1 -> convert_out4/1
  Gain1/1 -> convert_out1/1
  Shift Arithmetic2/1 -> Bitwise AND5/1
  Shift Arithmetic1/1 -> Bitwise AND5/2
  Bitwise AND5/1 -> Data Type Conversion1/1
  Data Type Conversion1/1 -> Mux2/2

== system SWC_HALOUT_type/run_SWC_HALOUT_Tx_5ms_sys/OUTP_AFTER/DID_list/uint16Touint8Array1 ==
  In1 : Inport
  Bitwise AND1 : simulink/Logic and Bit Operations/Bitwise Operator  logicop=AND  UseBitMask=on  BitMask=bin2dec('00000000000000000000000011111111')  BitMaskRealWorld=Stored Integer
  Bitwise AND2 : simulink/Logic and Bit Operations/Bitwise Operator  logicop=AND  UseBitMask=on  BitMask=bin2dec('00000000000000001111111100000000')  BitMaskRealWorld=Stored Integer
  Data Type Conversion1 : DataTypeConversion  OutDataTypeStr=uint8
  Data Type Conversion2 : DataTypeConversion  OutDataTypeStr=uint16
  Data Type Conversion5 : DataTypeConversion  OutDataTypeStr=uint8
  Mux2 : Mux  Inputs=2
  Shift Arithmetic39 : ArithShift  BitShiftNumber=8  BitShiftDirection=Right
  Out1 : Outport
  wires:
  Data Type Conversion1/1 -> Mux2/2
  Data Type Conversion5/1 -> Mux2/1
  Data Type Conversion2/1 -> Bitwise AND2/1, Bitwise AND1/1
  Bitwise AND2/1 -> Shift Arithmetic39/1
  Shift Arithmetic39/1 -> Data Type Conversion5/1
  In1/1 -> Data Type Conversion2/1
  Mux2/1 -> Out1/1
  Bitwise AND1/1 -> Data Type Conversion1/1

== system SWC_HALOUT_type/run_SWC_HALOUT_Tx_5ms_sys/OUTP_AFTER/DID_list/uint16Touint8Array10 ==
  In1 : Inport
  Bitwise AND1 : simulink/Logic and Bit Operations/Bitwise Operator  logicop=AND  UseBitMask=on  BitMask=bin2dec('00000000000000000000000011111111')  BitMaskRealWorld=Stored Integer
  Bitwise AND2 : simulink/Logic and Bit Operations/Bitwise Operator  logicop=AND  UseBitMask=on  BitMask=bin2dec('00000000000000001111111100000000')  BitMaskRealWorld=Stored Integer
  Data Type Conversion1 : DataTypeConversion  OutDataTypeStr=uint8
  Data Type Conversion2 : DataTypeConversion  OutDataTypeStr=uint16
  Data Type Conversion5 : DataTypeConversion  OutDataTypeStr=uint8
  Mux2 : Mux  Inputs=2
  Shift Arithmetic39 : ArithShift  BitShiftNumber=8  BitShiftDirection=Right
  Out1 : Outport
  wires:
  Data Type Conversion1/1 -> Mux2/2
  Data Type Conversion5/1 -> Mux2/1
  Data Type Conversion2/1 -> Bitwise AND2/1, Bitwise AND1/1
  Bitwise AND2/1 -> Shift Arithmetic39/1
  Shift Arithmetic39/1 -> Data Type Conversion5/1
  In1/1 -> Data Type Conversion2/1
  Mux2/1 -> Out1/1
  Bitwise AND1/1 -> Data Type Conversion1/1

== system SWC_HALOUT_type/run_SWC_HALOUT_Tx_5ms_sys/OUTP_AFTER/DID_list/uint16Touint8Array11 ==
  In1 : Inport
  Bitwise AND1 : simulink/Logic and Bit Operations/Bitwise Operator  logicop=AND  UseBitMask=on  BitMask=bin2dec('00000000000000000000000011111111')  BitMaskRealWorld=Stored Integer
  Bitwise AND2 : simulink/Logic and Bit Operations/Bitwise Operator  logicop=AND  UseBitMask=on  BitMask=bin2dec('00000000000000001111111100000000')  BitMaskRealWorld=Stored Integer
  Data Type Conversion1 : DataTypeConversion  OutDataTypeStr=uint8
  Data Type Conversion2 : DataTypeConversion  OutDataTypeStr=uint16
  Data Type Conversion5 : DataTypeConversion  OutDataTypeStr=uint8
  Mux2 : Mux  Inputs=2
  Shift Arithmetic39 : ArithShift  BitShiftNumber=8  BitShiftDirection=Right
  Out1 : Outport
  wires:
  Bitwise AND1/1 -> Data Type Conversion1/1
  Mux2/1 -> Out1/1
  In1/1 -> Data Type Conversion2/1
  Shift Arithmetic39/1 -> Data Type Conversion5/1
  Bitwise AND2/1 -> Shift Arithmetic39/1
  Data Type Conversion2/1 -> Bitwise AND1/1, Bitwise AND2/1
  Data Type Conversion5/1 -> Mux2/1
  Data Type Conversion1/1 -> Mux2/2

== system SWC_HALOUT_type/run_SWC_HALOUT_Tx_5ms_sys/OUTP_AFTER/DID_list/uint16Touint8Array12 ==
  In1 : Inport
  Bitwise AND1 : simulink/Logic and Bit Operations/Bitwise Operator  logicop=AND  UseBitMask=on  BitMask=bin2dec('00000000000000000000000011111111')  BitMaskRealWorld=Stored Integer
  Bitwise AND2 : simulink/Logic and Bit Operations/Bitwise Operator  logicop=AND  UseBitMask=on  BitMask=bin2dec('00000000000000001111111100000000')  BitMaskRealWorld=Stored Integer
  Data Type Conversion1 : DataTypeConversion  OutDataTypeStr=uint8
  Data Type Conversion2 : DataTypeConversion  OutDataTypeStr=uint16
  Data Type Conversion5 : DataTypeConversion  OutDataTypeStr=uint8
  Mux2 : Mux  Inputs=2
  Shift Arithmetic39 : ArithShift  BitShiftNumber=8  BitShiftDirection=Right
  Out1 : Outport
  wires:
  Data Type Conversion1/1 -> Mux2/2
  Data Type Conversion5/1 -> Mux2/1
  Data Type Conversion2/1 -> Bitwise AND2/1, Bitwise AND1/1
  Bitwise AND2/1 -> Shift Arithmetic39/1
  Shift Arithmetic39/1 -> Data Type Conversion5/1
  In1/1 -> Data Type Conversion2/1
  Mux2/1 -> Out1/1
  Bitwise AND1/1 -> Data Type Conversion1/1

== system SWC_HALOUT_type/run_SWC_HALOUT_Tx_5ms_sys/OUTP_AFTER/DID_list/uint16Touint8Array13 ==
  In1 : Inport
  Bitwise AND1 : simulink/Logic and Bit Operations/Bitwise Operator  logicop=AND  UseBitMask=on  BitMask=bin2dec('00000000000000000000000011111111')  BitMaskRealWorld=Stored Integer
  Bitwise AND2 : simulink/Logic and Bit Operations/Bitwise Operator  logicop=AND  UseBitMask=on  BitMask=bin2dec('00000000000000001111111100000000')  BitMaskRealWorld=Stored Integer
  Data Type Conversion1 : DataTypeConversion  OutDataTypeStr=uint8
  Data Type Conversion2 : DataTypeConversion  OutDataTypeStr=uint16
  Data Type Conversion5 : DataTypeConversion  OutDataTypeStr=uint8
  Mux2 : Mux  Inputs=2
  Shift Arithmetic39 : ArithShift  BitShiftNumber=8  BitShiftDirection=Right
  Out1 : Outport
  wires:
  Data Type Conversion1/1 -> Mux2/2
  Data Type Conversion5/1 -> Mux2/1
  Data Type Conversion2/1 -> Bitwise AND2/1, Bitwise AND1/1
  Bitwise AND2/1 -> Shift Arithmetic39/1
  Shift Arithmetic39/1 -> Data Type Conversion5/1
  In1/1 -> Data Type Conversion2/1
  Mux2/1 -> Out1/1
  Bitwise AND1/1 -> Data Type Conversion1/1

== system SWC_HALOUT_type/run_SWC_HALOUT_Tx_5ms_sys/OUTP_AFTER/DID_list/uint16Touint8Array14 ==
  In1 : Inport
  Bitwise AND1 : simulink/Logic and Bit Operations/Bitwise Operator  logicop=AND  UseBitMask=on  BitMask=bin2dec('00000000000000000000000011111111')  BitMaskRealWorld=Stored Integer
  Bitwise AND2 : simulink/Logic and Bit Operations/Bitwise Operator  logicop=AND  UseBitMask=on  BitMask=bin2dec('00000000000000001111111100000000')  BitMaskRealWorld=Stored Integer
  Data Type Conversion1 : DataTypeConversion  OutDataTypeStr=uint8
  Data Type Conversion2 : DataTypeConversion  OutDataTypeStr=uint16
  Data Type Conversion5 : DataTypeConversion  OutDataTypeStr=uint8
  Mux2 : Mux  Inputs=2
  Shift Arithmetic39 : ArithShift  BitShiftNumber=8  BitShiftDirection=Right
  Out1 : Outport
  wires:
  Bitwise AND1/1 -> Data Type Conversion1/1
  Mux2/1 -> Out1/1
  In1/1 -> Data Type Conversion2/1
  Shift Arithmetic39/1 -> Data Type Conversion5/1
  Bitwise AND2/1 -> Shift Arithmetic39/1
  Data Type Conversion2/1 -> Bitwise AND1/1, Bitwise AND2/1
  Data Type Conversion5/1 -> Mux2/1
  Data Type Conversion1/1 -> Mux2/2

== system SWC_HALOUT_type/run_SWC_HALOUT_Tx_5ms_sys/OUTP_AFTER/DID_list/uint16Touint8Array15 ==
  In1 : Inport
  Bitwise AND1 : simulink/Logic and Bit Operations/Bitwise Operator  logicop=AND  UseBitMask=on  BitMask=bin2dec('00000000000000000000000011111111')  BitMaskRealWorld=Stored Integer
  Bitwise AND2 : simulink/Logic and Bit Operations/Bitwise Operator  logicop=AND  UseBitMask=on  BitMask=bin2dec('00000000000000001111111100000000')  BitMaskRealWorld=Stored Integer
  Data Type Conversion1 : DataTypeConversion  OutDataTypeStr=uint8
  Data Type Conversion2 : DataTypeConversion  OutDataTypeStr=uint16
  Data Type Conversion5 : DataTypeConversion  OutDataTypeStr=uint8
  Mux2 : Mux  Inputs=2
  Shift Arithmetic39 : ArithShift  BitShiftNumber=8  BitShiftDirection=Right
  Out1 : Outport
  wires:
  Data Type Conversion1/1 -> Mux2/2
  Data Type Conversion5/1 -> Mux2/1
  Data Type Conversion2/1 -> Bitwise AND2/1, Bitwise AND1/1
  Bitwise AND2/1 -> Shift Arithmetic39/1
  Shift Arithmetic39/1 -> Data Type Conversion5/1
  In1/1 -> Data Type Conversion2/1
  Mux2/1 -> Out1/1
  Bitwise AND1/1 -> Data Type Conversion1/1

== system SWC_HALOUT_type/run_SWC_HALOUT_Tx_5ms_sys/OUTP_AFTER/DID_list/uint16Touint8Array16 ==
  In1 : Inport
  Bitwise AND1 : simulink/Logic and Bit Operations/Bitwise Operator  logicop=AND  UseBitMask=on  BitMask=bin2dec('00000000000000000000000011111111')  BitMaskRealWorld=Stored Integer
  Bitwise AND2 : simulink/Logic and Bit Operations/Bitwise Operator  logicop=AND  UseBitMask=on  BitMask=bin2dec('00000000000000001111111100000000')  BitMaskRealWorld=Stored Integer
  Data Type Conversion1 : DataTypeConversion  OutDataTypeStr=uint8
  Data Type Conversion2 : DataTypeConversion  OutDataTypeStr=uint16
  Data Type Conversion5 : DataTypeConversion  OutDataTypeStr=uint8
  Mux2 : Mux  Inputs=2
  Shift Arithmetic39 : ArithShift  BitShiftNumber=8  BitShiftDirection=Right
  Out1 : Outport
  wires:
  Data Type Conversion1/1 -> Mux2/2
  Data Type Conversion5/1 -> Mux2/1
  Data Type Conversion2/1 -> Bitwise AND2/1, Bitwise AND1/1
  Bitwise AND2/1 -> Shift Arithmetic39/1
  Shift Arithmetic39/1 -> Data Type Conversion5/1
  In1/1 -> Data Type Conversion2/1
  Mux2/1 -> Out1/1
  Bitwise AND1/1 -> Data Type Conversion1/1

== system SWC_HALOUT_type/run_SWC_HALOUT_Tx_5ms_sys/OUTP_AFTER/DID_list/uint16Touint8Array17 ==
  In1 : Inport
  Bitwise AND1 : simulink/Logic and Bit Operations/Bitwise Operator  logicop=AND  UseBitMask=on  BitMask=bin2dec('00000000000000000000000011111111')  BitMaskRealWorld=Stored Integer
  Bitwise AND2 : simulink/Logic and Bit Operations/Bitwise Operator  logicop=AND  UseBitMask=on  BitMask=bin2dec('00000000000000001111111100000000')  BitMaskRealWorld=Stored Integer
  Data Type Conversion1 : DataTypeConversion  OutDataTypeStr=uint8
  Data Type Conversion2 : DataTypeConversion  OutDataTypeStr=uint16
  Data Type Conversion5 : DataTypeConversion  OutDataTypeStr=uint8
  Mux2 : Mux  Inputs=2
  Shift Arithmetic39 : ArithShift  BitShiftNumber=8  BitShiftDirection=Right
  Out1 : Outport
  wires:
  Bitwise AND1/1 -> Data Type Conversion1/1
  Mux2/1 -> Out1/1
  In1/1 -> Data Type Conversion2/1
  Shift Arithmetic39/1 -> Data Type Conversion5/1
  Bitwise AND2/1 -> Shift Arithmetic39/1
  Data Type Conversion2/1 -> Bitwise AND1/1, Bitwise AND2/1
  Data Type Conversion5/1 -> Mux2/1
  Data Type Conversion1/1 -> Mux2/2

== system SWC_HALOUT_type/run_SWC_HALOUT_Tx_5ms_sys/OUTP_AFTER/DID_list/uint16Touint8Array18 ==
  In1 : Inport
  Bitwise AND1 : simulink/Logic and Bit Operations/Bitwise Operator  logicop=AND  UseBitMask=on  BitMask=bin2dec('00000000000000000000000011111111')  BitMaskRealWorld=Stored Integer
  Bitwise AND2 : simulink/Logic and Bit Operations/Bitwise Operator  logicop=AND  UseBitMask=on  BitMask=bin2dec('00000000000000001111111100000000')  BitMaskRealWorld=Stored Integer
  Data Type Conversion1 : DataTypeConversion  OutDataTypeStr=uint8
  Data Type Conversion2 : DataTypeConversion  OutDataTypeStr=uint16
  Data Type Conversion5 : DataTypeConversion  OutDataTypeStr=uint8
  Mux2 : Mux  Inputs=2
  Shift Arithmetic39 : ArithShift  BitShiftNumber=8  BitShiftDirection=Right
  Out1 : Outport
  wires:
  Data Type Conversion1/1 -> Mux2/2
  Data Type Conversion5/1 -> Mux2/1
  Data Type Conversion2/1 -> Bitwise AND2/1, Bitwise AND1/1
  Bitwise AND2/1 -> Shift Arithmetic39/1
  Shift Arithmetic39/1 -> Data Type Conversion5/1
  In1/1 -> Data Type Conversion2/1
  Mux2/1 -> Out1/1
  Bitwise AND1/1 -> Data Type Conversion1/1

== system SWC_HALOUT_type/run_SWC_HALOUT_Tx_5ms_sys/OUTP_AFTER/DID_list/uint16Touint8Array19 ==
  In1 : Inport
  Bitwise AND1 : simulink/Logic and Bit Operations/Bitwise Operator  logicop=AND  UseBitMask=on  BitMask=bin2dec('00000000000000000000000011111111')  BitMaskRealWorld=Stored Integer
  Bitwise AND2 : simulink/Logic and Bit Operations/Bitwise Operator  logicop=AND  UseBitMask=on  BitMask=bin2dec('00000000000000001111111100000000')  BitMaskRealWorld=Stored Integer
  Data Type Conversion1 : DataTypeConversion  OutDataTypeStr=uint8
  Data Type Conversion2 : DataTypeConversion  OutDataTypeStr=uint16
  Data Type Conversion5 : DataTypeConversion  OutDataTypeStr=uint8
  Mux2 : Mux  Inputs=2
  Shift Arithmetic39 : ArithShift  BitShiftNumber=8  BitShiftDirection=Right
  Out1 : Outport
  wires:
  Bitwise AND1/1 -> Data Type Conversion1/1
  Mux2/1 -> Out1/1
  In1/1 -> Data Type Conversion2/1
  Shift Arithmetic39/1 -> Data Type Conversion5/1
  Bitwise AND2/1 -> Shift Arithmetic39/1
  Data Type Conversion2/1 -> Bitwise AND1/1, Bitwise AND2/1
  Data Type Conversion5/1 -> Mux2/1
  Data Type Conversion1/1 -> Mux2/2

== system SWC_HALOUT_type/run_SWC_HALOUT_Tx_5ms_sys/OUTP_AFTER/DID_list/uint16Touint8Array2 ==
  In1 : Inport
  Bitwise AND1 : simulink/Logic and Bit Operations/Bitwise Operator  logicop=AND  UseBitMask=on  BitMask=bin2dec('00000000000000000000000011111111')  BitMaskRealWorld=Stored Integer
  Bitwise AND2 : simulink/Logic and Bit Operations/Bitwise Operator  logicop=AND  UseBitMask=on  BitMask=bin2dec('00000000000000001111111100000000')  BitMaskRealWorld=Stored Integer
  Data Type Conversion1 : DataTypeConversion  OutDataTypeStr=uint8
  Data Type Conversion2 : DataTypeConversion  OutDataTypeStr=uint16
  Data Type Conversion5 : DataTypeConversion  OutDataTypeStr=uint8
  Mux2 : Mux  Inputs=2
  Shift Arithmetic39 : ArithShift  BitShiftNumber=8  BitShiftDirection=Right
  Out1 : Outport
  wires:
  Bitwise AND1/1 -> Data Type Conversion1/1
  Mux2/1 -> Out1/1
  In1/1 -> Data Type Conversion2/1
  Shift Arithmetic39/1 -> Data Type Conversion5/1
  Bitwise AND2/1 -> Shift Arithmetic39/1
  Data Type Conversion2/1 -> Bitwise AND1/1, Bitwise AND2/1
  Data Type Conversion5/1 -> Mux2/1
  Data Type Conversion1/1 -> Mux2/2

== system SWC_HALOUT_type/run_SWC_HALOUT_Tx_5ms_sys/OUTP_AFTER/DID_list/uint16Touint8Array20 ==
  In1 : Inport
  Bitwise AND1 : simulink/Logic and Bit Operations/Bitwise Operator  logicop=AND  UseBitMask=on  BitMask=bin2dec('00000000000000000000000011111111')  BitMaskRealWorld=Stored Integer
  Bitwise AND2 : simulink/Logic and Bit Operations/Bitwise Operator  logicop=AND  UseBitMask=on  BitMask=bin2dec('00000000000000001111111100000000')  BitMaskRealWorld=Stored Integer
  Data Type Conversion1 : DataTypeConversion  OutDataTypeStr=uint8
  Data Type Conversion2 : DataTypeConversion  OutDataTypeStr=uint16
  Data Type Conversion5 : DataTypeConversion  OutDataTypeStr=uint8
  Mux2 : Mux  Inputs=2
  Shift Arithmetic39 : ArithShift  BitShiftNumber=8  BitShiftDirection=Right
  Out1 : Outport
  wires:
  Bitwise AND1/1 -> Data Type Conversion1/1
  Mux2/1 -> Out1/1
  In1/1 -> Data Type Conversion2/1
  Shift Arithmetic39/1 -> Data Type Conversion5/1
  Bitwise AND2/1 -> Shift Arithmetic39/1
  Data Type Conversion2/1 -> Bitwise AND1/1, Bitwise AND2/1
  Data Type Conversion5/1 -> Mux2/1
  Data Type Conversion1/1 -> Mux2/2

== system SWC_HALOUT_type/run_SWC_HALOUT_Tx_5ms_sys/OUTP_AFTER/DID_list/uint16Touint8Array21 ==
  In1 : Inport
  Bitwise AND1 : simulink/Logic and Bit Operations/Bitwise Operator  logicop=AND  UseBitMask=on  BitMask=bin2dec('00000000000000000000000011111111')  BitMaskRealWorld=Stored Integer
  Bitwise AND2 : simulink/Logic and Bit Operations/Bitwise Operator  logicop=AND  UseBitMask=on  BitMask=bin2dec('00000000000000001111111100000000')  BitMaskRealWorld=Stored Integer
  Data Type Conversion1 : DataTypeConversion  OutDataTypeStr=uint8
  Data Type Conversion2 : DataTypeConversion  OutDataTypeStr=uint16
  Data Type Conversion5 : DataTypeConversion  OutDataTypeStr=uint8
  Mux2 : Mux  Inputs=2
  Shift Arithmetic39 : ArithShift  BitShiftNumber=8  BitShiftDirection=Right
  Out1 : Outport
  wires:
  Data Type Conversion1/1 -> Mux2/2
  Data Type Conversion5/1 -> Mux2/1
  Data Type Conversion2/1 -> Bitwise AND2/1, Bitwise AND1/1
  Bitwise AND2/1 -> Shift Arithmetic39/1
  Shift Arithmetic39/1 -> Data Type Conversion5/1
  In1/1 -> Data Type Conversion2/1
  Mux2/1 -> Out1/1
  Bitwise AND1/1 -> Data Type Conversion1/1

== system SWC_HALOUT_type/run_SWC_HALOUT_Tx_5ms_sys/OUTP_AFTER/DID_list/uint16Touint8Array22 ==
  In1 : Inport
  Bitwise AND1 : simulink/Logic and Bit Operations/Bitwise Operator  logicop=AND  UseBitMask=on  BitMask=bin2dec('00000000000000000000000011111111')  BitMaskRealWorld=Stored Integer
  Bitwise AND2 : simulink/Logic and Bit Operations/Bitwise Operator  logicop=AND  UseBitMask=on  BitMask=bin2dec('00000000000000001111111100000000')  BitMaskRealWorld=Stored Integer
  Data Type Conversion1 : DataTypeConversion  OutDataTypeStr=uint8
  Data Type Conversion2 : DataTypeConversion  OutDataTypeStr=uint16
  Data Type Conversion5 : DataTypeConversion  OutDataTypeStr=uint8
  Mux2 : Mux  Inputs=2
  Shift Arithmetic39 : ArithShift  BitShiftNumber=8  BitShiftDirection=Right
  Out1 : Outport
  wires:
  Data Type Conversion1/1 -> Mux2/2
  Data Type Conversion5/1 -> Mux2/1
  Data Type Conversion2/1 -> Bitwise AND2/1, Bitwise AND1/1
  Bitwise AND2/1 -> Shift Arithmetic39/1
  Shift Arithmetic39/1 -> Data Type Conversion5/1
  In1/1 -> Data Type Conversion2/1
  Mux2/1 -> Out1/1
  Bitwise AND1/1 -> Data Type Conversion1/1

== system SWC_HALOUT_type/run_SWC_HALOUT_Tx_5ms_sys/OUTP_AFTER/DID_list/uint16Touint8Array23 ==
  In1 : Inport
  Bitwise AND1 : simulink/Logic and Bit Operations/Bitwise Operator  logicop=AND  UseBitMask=on  BitMask=bin2dec('00000000000000000000000011111111')  BitMaskRealWorld=Stored Integer
  Bitwise AND2 : simulink/Logic and Bit Operations/Bitwise Operator  logicop=AND  UseBitMask=on  BitMask=bin2dec('00000000000000001111111100000000')  BitMaskRealWorld=Stored Integer
  Data Type Conversion1 : DataTypeConversion  OutDataTypeStr=uint8
  Data Type Conversion2 : DataTypeConversion  OutDataTypeStr=uint16
  Data Type Conversion5 : DataTypeConversion  OutDataTypeStr=uint8
  Mux2 : Mux  Inputs=2
  Shift Arithmetic39 : ArithShift  BitShiftNumber=8  BitShiftDirection=Right
  Out1 : Outport
  wires:
  Bitwise AND1/1 -> Data Type Conversion1/1
  Mux2/1 -> Out1/1
  In1/1 -> Data Type Conversion2/1
  Shift Arithmetic39/1 -> Data Type Conversion5/1
  Bitwise AND2/1 -> Shift Arithmetic39/1
  Data Type Conversion2/1 -> Bitwise AND1/1, Bitwise AND2/1
  Data Type Conversion5/1 -> Mux2/1
  Data Type Conversion1/1 -> Mux2/2

== system SWC_HALOUT_type/run_SWC_HALOUT_Tx_5ms_sys/OUTP_AFTER/DID_list/uint16Touint8Array24 ==
  In1 : Inport
  Bitwise AND1 : simulink/Logic and Bit Operations/Bitwise Operator  logicop=AND  UseBitMask=on  BitMask=bin2dec('00000000000000000000000011111111')  BitMaskRealWorld=Stored Integer
  Bitwise AND2 : simulink/Logic and Bit Operations/Bitwise Operator  logicop=AND  UseBitMask=on  BitMask=bin2dec('00000000000000001111111100000000')  BitMaskRealWorld=Stored Integer
  Data Type Conversion1 : DataTypeConversion  OutDataTypeStr=uint8
  Data Type Conversion2 : DataTypeConversion  OutDataTypeStr=uint16
  Data Type Conversion5 : DataTypeConversion  OutDataTypeStr=uint8
  Mux2 : Mux  Inputs=2
  Shift Arithmetic39 : ArithShift  BitShiftNumber=8  BitShiftDirection=Right
  Out1 : Outport
  wires:
  Bitwise AND1/1 -> Data Type Conversion1/1
  Mux2/1 -> Out1/1
  In1/1 -> Data Type Conversion2/1
  Shift Arithmetic39/1 -> Data Type Conversion5/1
  Bitwise AND2/1 -> Shift Arithmetic39/1
  Data Type Conversion2/1 -> Bitwise AND1/1, Bitwise AND2/1
  Data Type Conversion5/1 -> Mux2/1
  Data Type Conversion1/1 -> Mux2/2

== system SWC_HALOUT_type/run_SWC_HALOUT_Tx_5ms_sys/OUTP_AFTER/DID_list/uint16Touint8Array25 ==
  In1 : Inport
  Bitwise AND1 : simulink/Logic and Bit Operations/Bitwise Operator  logicop=AND  UseBitMask=on  BitMask=bin2dec('00000000000000000000000011111111')  BitMaskRealWorld=Stored Integer
  Bitwise AND2 : simulink/Logic and Bit Operations/Bitwise Operator  logicop=AND  UseBitMask=on  BitMask=bin2dec('00000000000000001111111100000000')  BitMaskRealWorld=Stored Integer
  Data Type Conversion1 : DataTypeConversion  OutDataTypeStr=uint8
  Data Type Conversion2 : DataTypeConversion  OutDataTypeStr=uint16
  Data Type Conversion5 : DataTypeConversion  OutDataTypeStr=uint8
  Mux2 : Mux  Inputs=2
  Shift Arithmetic39 : ArithShift  BitShiftNumber=8  BitShiftDirection=Right
  Out1 : Outport
  wires:
  Data Type Conversion1/1 -> Mux2/2
  Data Type Conversion5/1 -> Mux2/1
  Data Type Conversion2/1 -> Bitwise AND2/1, Bitwise AND1/1
  Bitwise AND2/1 -> Shift Arithmetic39/1
  Shift Arithmetic39/1 -> Data Type Conversion5/1
  In1/1 -> Data Type Conversion2/1
  Mux2/1 -> Out1/1
  Bitwise AND1/1 -> Data Type Conversion1/1

== system SWC_HALOUT_type/run_SWC_HALOUT_Tx_5ms_sys/OUTP_AFTER/DID_list/uint16Touint8Array26 ==
  In1 : Inport
  Bitwise AND1 : simulink/Logic and Bit Operations/Bitwise Operator  logicop=AND  UseBitMask=on  BitMask=bin2dec('00000000000000000000000011111111')  BitMaskRealWorld=Stored Integer
  Bitwise AND2 : simulink/Logic and Bit Operations/Bitwise Operator  logicop=AND  UseBitMask=on  BitMask=bin2dec('00000000000000001111111100000000')  BitMaskRealWorld=Stored Integer
  Data Type Conversion1 : DataTypeConversion  OutDataTypeStr=uint8
  Data Type Conversion2 : DataTypeConversion  OutDataTypeStr=uint16
  Data Type Conversion5 : DataTypeConversion  OutDataTypeStr=uint8
  Mux2 : Mux  Inputs=2
  Shift Arithmetic39 : ArithShift  BitShiftNumber=8  BitShiftDirection=Right
  Out1 : Outport
  wires:
  Bitwise AND1/1 -> Data Type Conversion1/1
  Mux2/1 -> Out1/1
  In1/1 -> Data Type Conversion2/1
  Shift Arithmetic39/1 -> Data Type Conversion5/1
  Bitwise AND2/1 -> Shift Arithmetic39/1
  Data Type Conversion2/1 -> Bitwise AND1/1, Bitwise AND2/1
  Data Type Conversion5/1 -> Mux2/1
  Data Type Conversion1/1 -> Mux2/2
